simulink model "SteerCtrl_V1_1"  (R2018a)
settings: Solver=FixedStepDiscrete  StartTime=0.0  StopTime=10.0  FixedStep=sampletime  RelTol=1e-3  EnableMultiTasking=on
PreLoadFcn:
  | SteerCtrl_V1_BusInfo
libraries: simulink x2
settings Model: Creator=IAEC nishito  LastModifiedBy=E00026
settings DataIOCC: LimitDataPoints=on  SaveFormat=Array  SignalLoggingSaveFormat=ModelDataLogs  SaveOutput=off
settings OptimizationCC: DefaultParameterBehavior=Inlined  ExpressionDepthLimit=2147483647  LifeSpan=inf
settings DebuggingCC: UnderspecifiedInitializationDetection=Classic  MergeDetectMultiDrivingBlocksExec=none  SolverPrmCheckMsg=warning  FcnCallInpInsideContextMsg=warning  StateNameClashWarn=warning  SFUnexpectedBacktrackingDiag=warning  SFNoUnconditionalDefaultTransitionDiag=warning  SFExecutionAtInitializationDiag=none
settings HardwareCC: ProdBitPerPointer=32  ProdBitPerSizeT=32  ProdBitPerPtrDiffT=32  ProdLargestAtomicFloat=None  ProdIntDivRoundTo=Undefined  ProdEndianess=Unspecified  ProdWordSize=32  ProdHWDeviceType=32-bit Generic
settings ModelReferenceCC: UpdateModelReferenceTargets=IfOutOfDate  PropagateSignalLabelsOutOfModel=off
settings CodeAppCC: StateflowObjectComments=on
settings GRTTargetCC: TargetLangStandard=C89/C90 (ANSI)  GeneratePreprocessorConditionals=Disable all  CombineOutputUpdateFcns=off  GRTInterface=on
settings ConfigComp: CovMetricSettings=dw  CovHtmlReporting=on  CovSaveCumulativeToWorkspaceVar=on  CovSaveSingleToWorkspaceVar=on  CovExternalEMLEnable=off  CovSFcnEnable=off

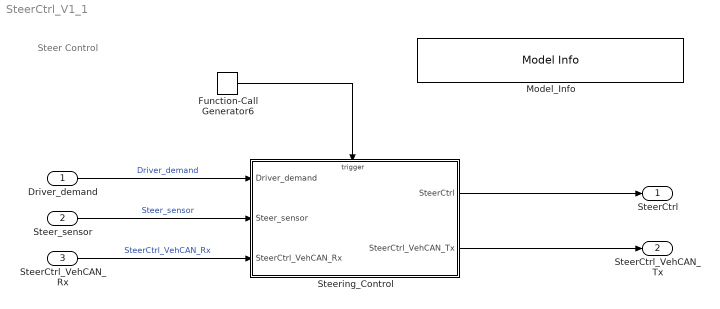
== system SteerCtrl_V1_1 ==
  note: Steer Control
  Driver_demand : Inport  OutDataTypeStr=Bus: Driver_demand_Bus
      settings: AttributesFormatString=<%<OutDataTypeStr>>
  Steer_sensor : Inport  Port=2  OutDataTypeStr=Bus: Steer_sensor_Bus
      settings: AttributesFormatString=<%<OutDataTypeStr>>
  SteerCtrl_VehCAN_Rx : Inport  Port=3  OutDataTypeStr=Bus: SteerCtrl_VehCAN_Rx_Bus
      settings: AttributesFormatString=<%<OutDataTypeStr>>
  Function-Call Generator6 : simulink/Ports & Subsystems/Function-Call Generator  sample_time=0.05  numberOfIterations=1
      settings: AttributesFormatString=<sample_time=%<sample_time>>
  Model_Info : simulink/Model-Wide Utilities/Model Info  Frame=on  DisplayStringWithTags=|  HorizontalTextAlignment=Left  LeftAlignmentValue=0.02
      | Version  %<ModelVersion>
      | LastModifided by %<LastModifiedBy>  Date %<LastModificationDate>
      | Description  %<Description>
  Steering_Control : Subsystem
  SteerCtrl : Outport  OutDataTypeStr=Bus: SteerCtrl_Bus
      settings: AttributesFormatString=<%<OutDataTypeStr>>
  SteerCtrl_VehCAN_Tx : Outport  Port=2  OutDataTypeStr=Bus: SteerCtrl_VehCAN_Tx_Bus
      settings: AttributesFormatString=<%<OutDataTypeStr>>
  wires:
  Steering_Control/2(SteerCtrl_VehCAN_Tx) -> SteerCtrl_VehCAN_Tx/1
  SteerCtrl_VehCAN_Rx/1 -> Steering_Control/3(SteerCtrl_VehCAN_Rx)  "SteerCtrl_VehCAN_Rx"
  Driver_demand/1 -> Steering_Control/1(Driver_demand)  "Driver_demand"
  Steering_Control/1(SteerCtrl) -> SteerCtrl/1
  Steer_sensor/1 -> Steering_Control/2(Steer_sensor)  "Steer_sensor"
  Function-Call Generator6/1 -> Steering_Control/Trigger

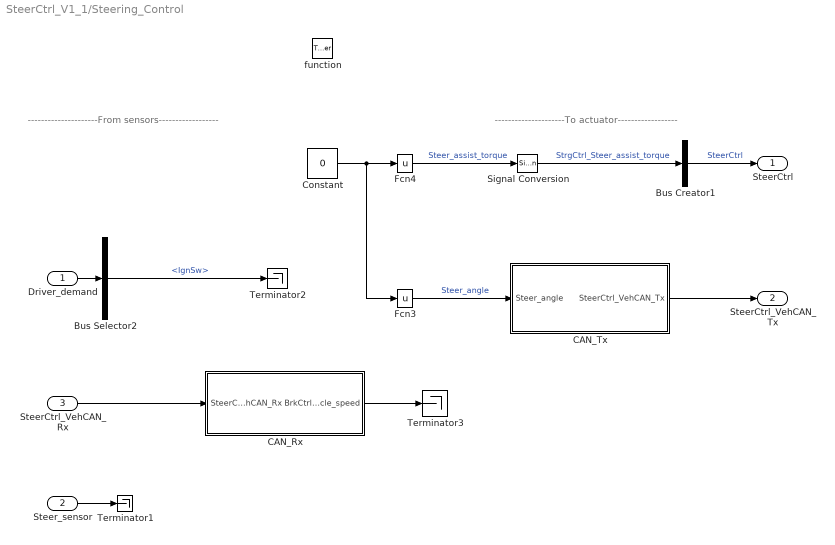
== system SteerCtrl_V1_1/Steering_Control ==
  note: ---------------------From sensors------------------
  note: ---------------------To actuator------------------
  Driver_demand : Inport
  Steer_sensor : Inport  Port=2
  SteerCtrl_VehCAN_Rx : Inport  Port=3
  function : TriggerPort  TriggerType=function-call  VariantControl=Variant
  Bus Creator1 : BusCreator  Inputs=1  OutDataTypeStr=Bus: SteerCtrl_Bus
      settings: AttributesFormatString=<%<OutDataTypeStr>>
  Bus Selector2 : BusSelector  OutputSignals=IgnSw
  CAN_Rx : Subsystem
  CAN_Tx : Subsystem
  Constant : Constant  Value=0
  Fcn3 : Fcn  Expr=u
  Fcn4 : Fcn  Expr=u
  Signal Conversion : SignalConversion  OverrideOpt=off
  Terminator1 : Terminator
  Terminator2 : Terminator
  Terminator3 : Terminator
  SteerCtrl : Outport
  SteerCtrl_VehCAN_Tx : Outport  Port=2
  wires:
  Fcn4/1 -> Signal Conversion/1  "Steer_assist_torque"
  Driver_demand/1 -> Bus Selector2/1
  Bus Creator1/1 -> SteerCtrl/1  "SteerCtrl"
  SteerCtrl_VehCAN_Rx/1 -> CAN_Rx/1(SteerCtrl_VehCAN_Rx)
  Constant/1 -> Fcn3/1, Fcn4/1
  Bus Selector2/1 -> Terminator2/1  "<IgnSw>"
  Steer_sensor/1 -> Terminator1/1
  Signal Conversion/1 -> Bus Creator1/1  "StrgCtrl_Steer_assist_torque"
  CAN_Rx/1(BrkCtrl_Vehicle_speed) -> Terminator3/1
  Fcn3/1 -> CAN_Tx/1(Steer_angle)  "Steer_angle"
  CAN_Tx/1(SteerCtrl_VehCAN_Tx) -> SteerCtrl_VehCAN_Tx/1

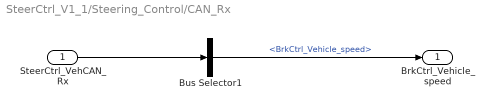
== system SteerCtrl_V1_1/Steering_Control/CAN_Rx ==
  SteerCtrl_VehCAN_Rx : Inport
  Bus Selector1 : BusSelector  OutputSignals=BrkCtrl_Vehicle_speed
  BrkCtrl_Vehicle_speed : Outport
  wires:
  Bus Selector1/1 -> BrkCtrl_Vehicle_speed/1  "<BrkCtrl_Vehicle_speed>"
  SteerCtrl_VehCAN_Rx/1 -> Bus Selector1/1

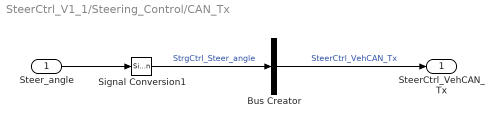
== system SteerCtrl_V1_1/Steering_Control/CAN_Tx ==
  Steer_angle : Inport
  Bus Creator : BusCreator  Inputs=1  OutDataTypeStr=Bus: SteerCtrl_VehCAN_Tx_Bus
      settings: AttributesFormatString=<%<OutDataTypeStr>>
  Signal Conversion1 : SignalConversion  OverrideOpt=off
  SteerCtrl_VehCAN_Tx : Outport
  wires:
  Signal Conversion1/1 -> Bus Creator/1  "StrgCtrl_Steer_angle"
  Bus Creator/1 -> SteerCtrl_VehCAN_Tx/1  "SteerCtrl_VehCAN_Tx"
  Steer_angle/1 -> Signal Conversion1/1
